simulink library "ESTS_UOD_AgrVSideSlipVehPreproc"  (R2022a)
settings: Solver=VariableStepAuto  StartTime=0.0  StopTime=10.0  RelTol=1e-3
undefined symbols (not defined in the file or in its folder): ESTS_UOD_p_Tau_s, ESTS_UOSD_c_TiSample_s
libraries: VUT_lib x2
settings Model: Creator=blatak  LastModifiedBy=blatak

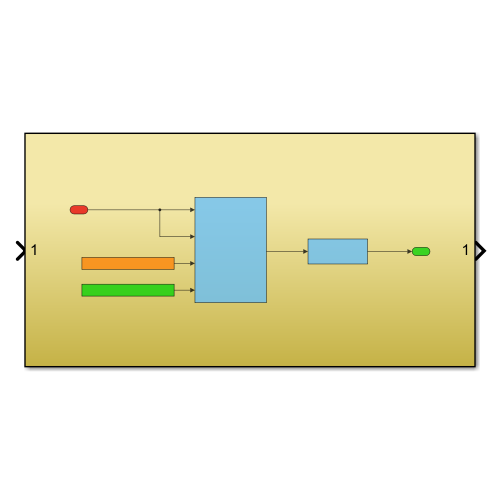
[thumbnail: Simulink's stored preview of the top-level diagram]
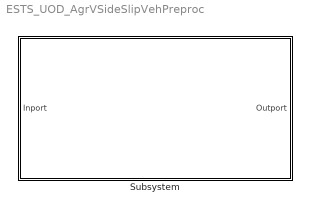
== system ESTS_UOD_AgrVSideSlipVehPreproc ==
  Subsystem : Subsystem

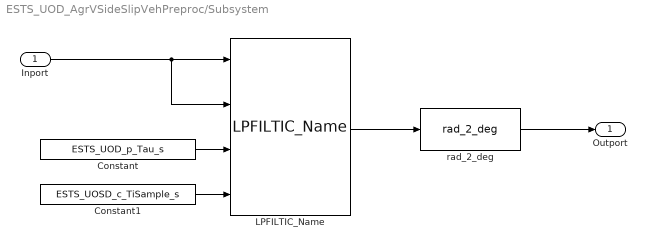
== system ESTS_UOD_AgrVSideSlipVehPreproc/Subsystem ==
  Inport : Inport
  Constant : Constant  Value=ESTS_UOD_p_Tau_s
  Constant1 : Constant  Value=ESTS_UOSD_c_TiSample_s
  LPFILTIC_Name : VUT_lib/LPFILTIC_Name  SystemSampleTime=-1  VariantActivationTime=update diagram  Latency=0  AutoFrameSizeCalculation=off
  rad_2_deg : VUT_lib/rad_2_deg  SystemSampleTime=-1  VariantActivationTime=update diagram  Latency=0  AutoFrameSizeCalculation=off
  Outport : Outport
  wires:
  LPFILTIC_Name/1 -> rad_2_deg/1
  rad_2_deg/1 -> Outport/1
  Inport/1 -> LPFILTIC_Name/2, LPFILTIC_Name/1
  Constant1/1 -> LPFILTIC_Name/4
  Constant/1 -> LPFILTIC_Name/3
